simulink model "TCS_new"  (R2023b)
settings: Solver=ode5  StartTime=0.0  StopTime=10  FixedStep=.001  RelTol=1e-3
libraries: slpidlib x1
settings Model: Creator=ibaad  LastModifiedBy=ajame
settings DebuggingCC: AlgebraicLoopMsg=none

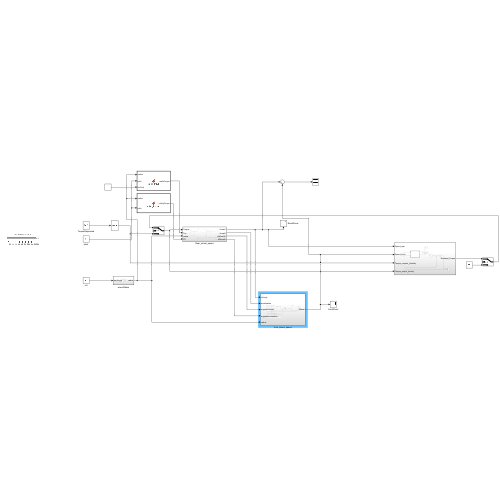
[thumbnail: Simulink's stored preview of the top-level diagram]
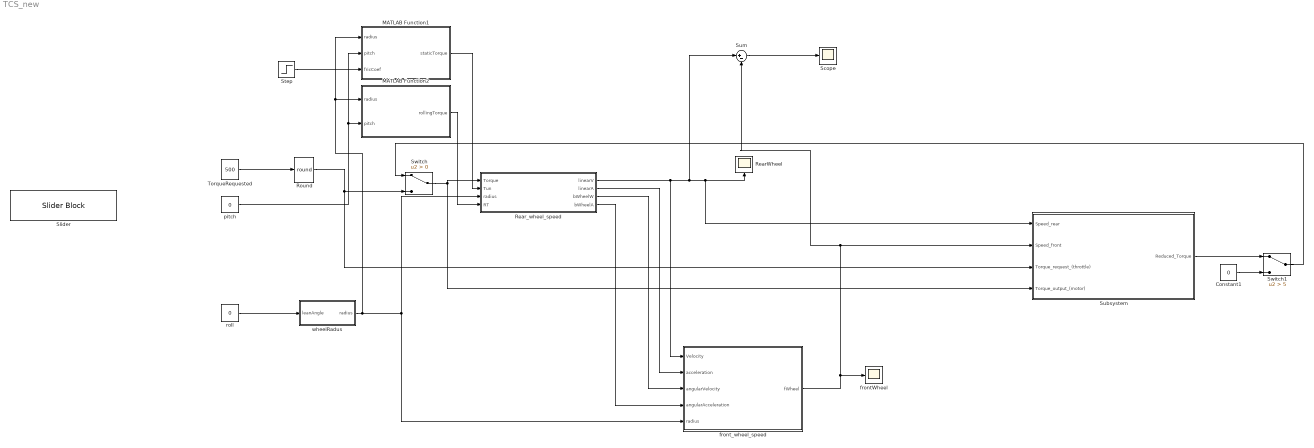
== system TCS_new ==
  Constant1 : Constant  Value=0
  MATLAB Function1 : MATLAB Function  TreatAsAtomicUnit=on
  MATLAB Function2 : MATLAB Function  TreatAsAtomicUnit=on
  RearWheel : Scope
  Rear_wheel_speed : Subsystem
  Round : Rounding  Operator=round
  Scope : Scope
  Slider : SliderBlock  ScaleMax=500
  Step : Step  Time=5  Before=1.12  SampleTime=0
  Subsystem : Subsystem
  Sum : Sum  Inputs=|+-
  Switch : Switch  Criteria=u2 > Threshold  SaturateOnIntegerOverflow=off  InputSameDT=off
  Switch1 : Switch  Criteria=u2 > Threshold  Threshold=5  SaturateOnIntegerOverflow=off  InputSameDT=off
  TorqueRequested : Constant  Value=500
  frontWheel : Scope
  front_wheel_speed : Subsystem
  pitch : Constant  Value=0
  roll : Constant  Value=0
  wheelRadus : Subsystem
  wires:
  TorqueRequested/1 -> Round/1
  Switch/1 -> Rear_wheel_speed/1(Torque), Subsystem/4(Torque_output_(motor))
  Round/1 -> Switch/3, Subsystem/3(Torque_request_(throttle))
  roll/1 -> wheelRadus/1(leanAngle)
  Subsystem/1(Reduced_Torque) -> Switch1/1
  Constant1/1 -> Switch1/3
  Rear_wheel_speed/1(linearV) -> Sum/1, RearWheel/1, Subsystem/1(Speed_rear), front_wheel_speed/1(Velocity)
  MATLAB Function1/1(staticTorque) -> Rear_wheel_speed/2(Tun)
  MATLAB Function2/1(rollingTorque) -> Rear_wheel_speed/4(RT)
  Switch1/1 -> Switch/1
  pitch/1 -> MATLAB Function1/2(pitch), MATLAB Function2/2(pitch)
  wheelRadus/1(radius) -> MATLAB Function2/1(radius), MATLAB Function1/1(radius), front_wheel_speed/5(radius), Rear_wheel_speed/3(radius)
  Rear_wheel_speed/2(linearA) -> front_wheel_speed/2(acceleration)
  Rear_wheel_speed/3(bWheelW) -> front_wheel_speed/3(angularVelocity)
  Rear_wheel_speed/4(bWheelA) -> front_wheel_speed/4(angularAcceleration)
  Step/1 -> MATLAB Function1/3(fricCoef)
  front_wheel_speed/1(fWheel) -> Subsystem/2(Speed_front), Sum/2, frontWheel/1
  Sum/1 -> Scope/1

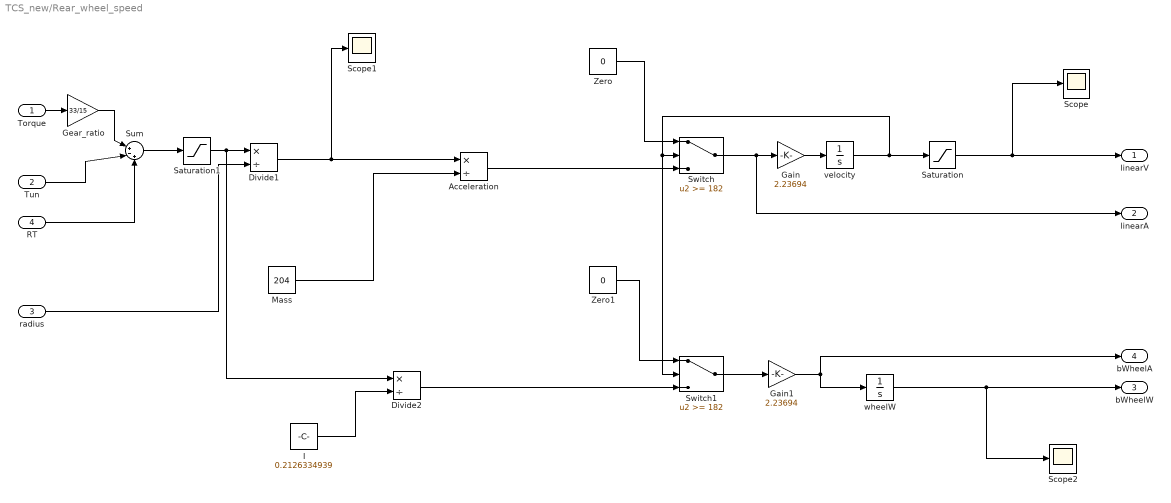
== system TCS_new/Rear_wheel_speed ==
  Torque : Inport
  Tun : Inport  Port=2
  radius : Inport  Port=3
  RT : Inport  Port=4
  Acceleration : Product  Inputs=*/
  Divide1 : Product  Inputs=*/
  Divide2 : Product  Inputs=*/
  Gain : Gain  Gain=2.23694
  Gain1 : Gain  Gain=2.23694
  Gear_ratio : Gain  Gain=33/15
  I : Constant  Value=0.2126334939
  Mass : Constant  Value=204
  Saturation : Saturate  UpperLimit=182  LowerLimit=0
  Saturation1 : Saturate  UpperLimit=inf  LowerLimit=0
  Scope : Scope
  Scope1 : Scope
  Scope2 : Scope
  Sum : Sum  Inputs=|+-+
  Switch : Switch  Threshold=182  SaturateOnIntegerOverflow=off  InputSameDT=off
  Switch1 : Switch  Threshold=182  SaturateOnIntegerOverflow=off  InputSameDT=off
  Zero : Constant  Value=0  OutDataTypeStr=Inherit: Inherit via back propagation
  Zero1 : Constant  Value=0  OutDataTypeStr=Inherit: Inherit via back propagation
  velocity : Integrator
  wheelW : Integrator
  linearV : Outport
  linearA : Outport  Port=2
  bWheelW : Outport  Port=3
  bWheelA : Outport  Port=4
  wires:
  Acceleration/1 -> Switch/3
  Torque/1 -> Gear_ratio/1
  Gear_ratio/1 -> Sum/1
  Divide1/1 -> Scope1/1, Acceleration/1
  radius/1 -> Divide1/2
  Tun/1 -> Sum/2
  Sum/1 -> Saturation1/1
  Saturation1/1 -> Divide2/1, Divide1/1
  RT/1 -> Sum/3
  Saturation/1 -> Scope/1, linearV/1
  Mass/1 -> Acceleration/2
  Switch/1 -> Gain/1, linearA/1
  Zero/1 -> Switch/1
  I/1 -> Divide2/2
  Zero1/1 -> Switch1/1
  Divide2/1 -> Switch1/3
  Switch1/1 -> Gain1/1
  wheelW/1 -> Scope2/1, bWheelW/1
  Gain/1 -> velocity/1
  velocity/1 -> Switch1/2, Switch/2, Saturation/1
  Gain1/1 -> wheelW/1, bWheelA/1

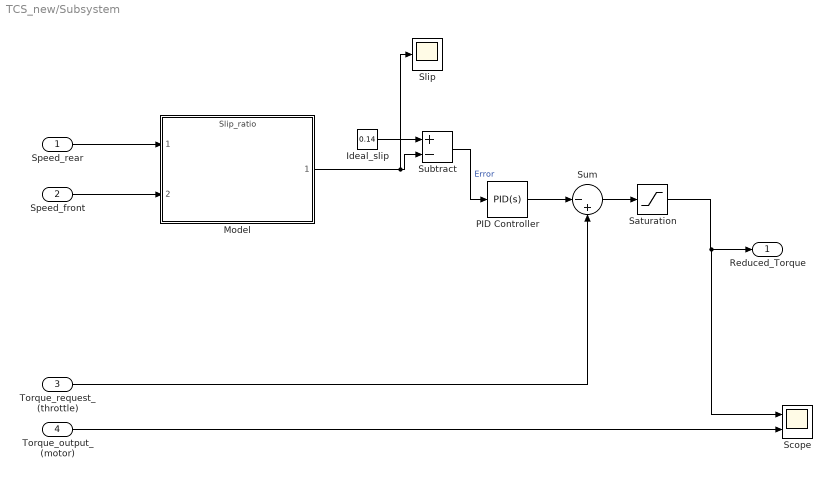
== system TCS_new/Subsystem ==
  Speed_rear : Inport
  Speed_front : Inport  Port=2
  Torque_request_(throttle) : Inport  Port=3
  Torque_output_(motor) : Inport  Port=4
  Ideal_slip : Constant  Value=0.14
  Model : ModelReference  ModelNameDialog=Slip_ratio.slx  SimulationMode=Normal  ModelReferenceVersion=2.2
  PID Controller : slpidlib/PID Controller  Controller=PID  Form=Parallel  TimeDomain=Continuous-time  UseExternalTs=off  SampleTime=-1  IntegratorMethod=Forward Euler  FilterMethod=Forward Euler  ControllerParametersSource=internal  P=1  I=0  UseKiTs=off  D=0  N=100  UseFilter=on  TunerSelectOption=Transfer Function Based (PID Tuner App)  InitialConditionSource=internal  InitialConditionForIntegrator=0  InitialConditionForFilter=0  DifferentiatorICPrevScaledInput=0  ExternalReset=none  TrackingMode=off  Kt=1  LimitOutput=off  SatLimitsSource=internal  UpperSaturationLimit=inf  LowerSaturationLimit=-inf  LinearizeAsGain=on  AntiWindupMode=none  Kb=1  LimitIntegrator=off  UpperIntegratorSaturationLimit=inf  LowerIntegratorSaturationLimit=-inf  POutMin=[]  POutMax=[]  IOutMin=[]  IOutMax=[]  DOutMin=[]  DOutMax=[]  NOutMin=[]  NOutMax=[]  SumOutMin=[]  SumOutMax=[]  SaturationOutMin=[]  SaturationOutMax=[]  PParamMin=[]  PParamMax=[]  IParamMin=[]  IParamMax=[]  DParamMin=[]  DParamMax=[]  NParamMin=[]  NParamMax=[]  KbParamMin=[]  KbParamMax=[]  KtParamMin=[]  KtParamMax=[]  KbOutMin=[]  KbOutMax=[]  KtOutMin=[]  KtOutMax=[]  IntegratorOutMin=[]  IntegratorOutMax=[]  FilterOutMin=[]  FilterOutMax=[]  SumI1OutMin=[]  SumI1OutMax=[]  SumI2OutMin=[]  SumI2OutMax=[]  SumI3OutMin=[]  SumI3OutMax=[]  SumI4OutMin=[]  SumI4OutMax=[]  SumDOutMin=[]  SumDOutMax=[]  DifferentiatorOutMin=[]  DifferentiatorOutMax=[]  FilterDiffOutCoefMin=[]  FilterDiffOutCoefMax=[]  ReciprocalOutMin=[]  ReciprocalOutMax=[]  SumDenOutMin=[]  SumDenOutMax=[]  SumNumOutMin=[]  SumNumOutMax=[]  DivideOutMin=[]  DivideOutMax=[]  UdiffTsProdOutMin=[]  UdiffTsProdOutMax=[]  NTsProdOutMin=[]  NTsProdOutMax=[]  UintegralTsProdOutMin=[]  UintegralTsProdOutMax=[]  UngainTsProdOutMin=[]  UngainTsProdOutMax=[]  ClampingZeroOutDataTypeStr=Inherit: Inherit via back propagation  ClampingZeroOutMin=[]  ClampingZeroOutMax=[]  FilterDenConstantOutDataTypeStr=Inherit: Inherit via back propagation  FilterDenConstantOutMin=[]  FilterDenConstantOutMax=[]  PCopyOutDataTypeStr=Inherit: Inherit via back propagation  PCopyOutMin=[]  PCopyOutMax=[]  NCopyOutDataTypeStr=Inherit: Inherit via back propagation  NCopyOutMin=[]  NCopyOutMax=[]  IntegratorContinuousStateAttributes=''  IntegratorStateMustResolveToSignalObject=off  IntegratorRTWStateStorageClass=Auto  FilterContinuousStateAttributes=''  FilterStateMustResolveToSignalObject=off  FilterRTWStateStorageClass=Auto  ParallelPVariant=InternalParameters  IdealPVariant=Disabled  IVariant=InternalParameters  DVariant=InternalParameters  IntegratorVariant=Continuous  SatVariant=Disabled  AWVariant=Passthrough  PCopyVariant=Disabled  TRVariant=Disabled  FdbkBlocksVariant=Forward  IdealPFdbkVariant=Disabled  SatFdbkVariant=Disabled  DerivativeFilterVariant=ContFilter  NVariant=InternalParameters  NCopyVariant=Disabled  FilterICVariant=InternalICsFilter  IntegratorICVariant=InternalICs  ExternalResetVariant=Disabled  TRSumVariant=Passthrough  SumFdbkVariant=Disabled  SumVariant=Sum_PID  TsampFilterVariant=InternalTs  TsampNgainVariant=Passthrough  TsampIntegralVariant=Disabled_SignalSpec  ExternalSaturationOutDataTypeStr=Inherit: Same as second input
  Saturation : Saturate  UpperLimit=320  LowerLimit=0
  Scope : Scope  NumInputPorts=2
  Slip : Scope
  Subtract : Sum  Inputs=+-
  Sum : Sum  Inputs=|-+
  Reduced_Torque : Outport
  wires:
  Speed_front/1 -> Model/2
  Speed_rear/1 -> Model/1
  Ideal_slip/1 -> Subtract/1
  Model/1 -> Slip/1, Subtract/2
  Subtract/1 -> PID Controller/1  "Error"
  PID Controller/1 -> Sum/1
  Torque_request_(throttle)/1 -> Sum/2
  Sum/1 -> Saturation/1
  Saturation/1 -> Scope/1, Reduced_Torque/1
  Torque_output_(motor)/1 -> Scope/2

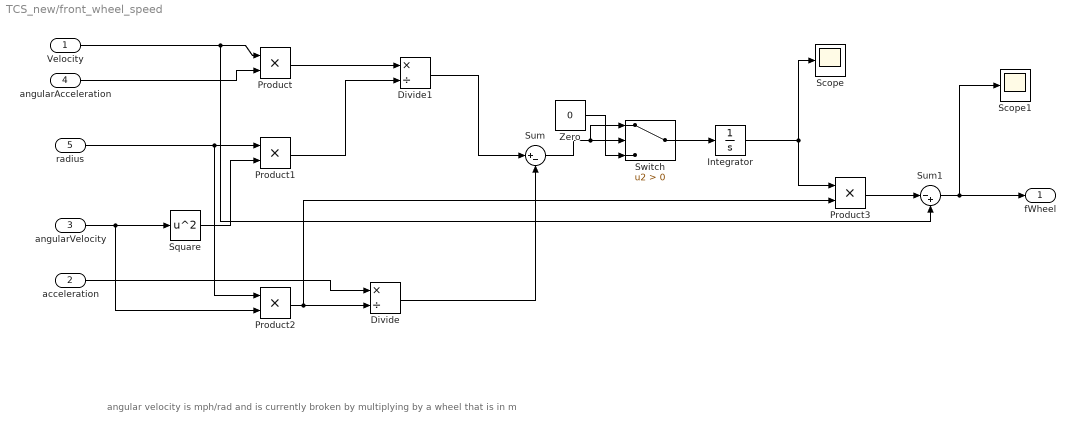
== system TCS_new/front_wheel_speed ==
  note: angular velocity is mph/rad and is currently broken by multiplying by a wheel that is in m
  Velocity : Inport
  acceleration : Inport  Port=2
  angularVelocity : Inport  Port=3
  angularAcceleration : Inport  Port=4
  radius : Inport  Port=5
  Divide : Product  Inputs=*/
  Divide1 : Product  Inputs=*/
  Integrator : Integrator
  Product{,1..3} (4 alike) : Product
  Scope : Scope
  Scope1 : Scope
  Square : Math  Operator=square
  Sum : Sum  Inputs=|+-
  Sum1 : Sum  Inputs=|-+
  Switch : Switch  Criteria=u2 > Threshold  SaturateOnIntegerOverflow=off  InputSameDT=off
  Zero : Constant  Value=0  OutDataTypeStr=Inherit: Inherit via back propagation
  fWheel : Outport
  wires:
  angularAcceleration/1 -> Product/2
  radius/1 -> Product2/1, Product1/1
  Square/1 -> Product1/2
  angularVelocity/1 -> Product2/2, Square/1
  acceleration/1 -> Divide/1
  Product1/1 -> Divide1/2
  Product/1 -> Divide1/1
  Divide1/1 -> Sum/1
  Divide/1 -> Sum/2
  Sum/1 -> Switch/1, Switch/2
  Switch/1 -> Integrator/1
  Zero/1 -> Switch/3
  Integrator/1 -> Product3/1, Scope/1
  Product3/1 -> Sum1/1
  Sum1/1 -> Scope1/1, fWheel/1
  Velocity/1 -> Sum1/2, Product/1
  Product2/1 -> Product3/2, Divide/2

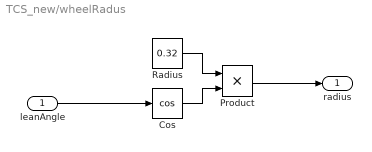
== system TCS_new/wheelRadus ==
  leanAngle : Inport
  Cos : Trigonometry  Operator=cos
  Product : Product
  Radius : Constant  Value=0.32
  radius : Outport
  wires:
  leanAngle/1 -> Cos/1
  Radius/1 -> Product/1
  Cos/1 -> Product/2
  Product/1 -> radius/1

== matlab function TCS_new/MATLAB Function2 ==
  data: rollingTorque output; radius input; pitch input
function rollingTorque = rollingTorque(radius,pitch)
    % TCS_ACTIVE Summary of this function goes here
    weightBike = 1989.5; %in N
    weightDistribution = .5; % fore and aft
    tire = .32; % in m
    
    Tyre_radius = radius;
    fricCoef = 0.02;
    Fn = weightBike*weightDistribution*cos(pitch);
    rollingTorque = ((fricCoef * Fn) * Tyre_radius);
end

== matlab function TCS_new/MATLAB Function1 ==
  data: staticTorque output; radius input; pitch input; fricCoef input
function staticTorque = staticTorque(radius,pitch,fricCoef)
    % TCS_ACTIVE Summary of this function goes here

    e = exp(1); % Mathematical constant e
    % Friction curve as a function of slip ratio
    c1 = 1.2801; % Coef for dry asphalt

    weightBike = 1989.5; %in N
    weightDistribution = .5; % fore and aft
    tire = .32; % in m
    
    Tyre_radius = radius;
    %fricCoef = c1;
    Fn = weightBike*weightDistribution*cos(pitch);
    staticTorque = ((fricCoef * Fn) * Tyre_radius);
end
